simulink model "modelo_mpc_sem_restricao"  (R2018b)
settings: Solver=VariableStepAuto  StartTime=0.0  StopTime=100  RelTol=1e-3
values from neighbouring files (symbols this model uses):
  A = [0 1 0 0 ... (first row only)    [dadosBallBeam.m]    (also in dadosTanqueQuatro.m = [-1/T1 0 A3/(A1*T3) 0; tanqueQuatroLinearizacao.m = double(subs(As,{h1,h2,h3,h4,v1,v2},{h10,h20,h30,h40,v10,v20})
  A1 = 28    [dadosTanqueQuatro.m]    (also in tanqueQuatroLinearizacao.m)
  a1 = 0.071    [dadosTanqueQuatro.m]    (also in tanqueQuatroLinearizacao.m)
  A2 = 32    [dadosTanqueQuatro.m]    (also in tanqueQuatroLinearizacao.m)
  a2 = 0.057    [dadosTanqueQuatro.m]    (also in tanqueQuatroLinearizacao.m)
  a3 = 0.071    [dadosTanqueQuatro.m]    (also in tanqueQuatroLinearizacao.m)
  A3 = 28    [dadosTanqueQuatro.m]    (also in tanqueQuatroLinearizacao.m)
  a4 = 0.057    [dadosTanqueQuatro.m]    (also in tanqueQuatroLinearizacao.m)
  A4 = 32    [dadosTanqueQuatro.m]    (also in tanqueQuatroLinearizacao.m)
  B = [0 0 0 1]'    [dadosBallBeam.m]    (also in dadosTanqueQuatro.m = [(y1*k1)/A1 0; tanqueQuatroLinearizacao.m = double(subs(Bs,{h1,h2,h3,h4,v1,v2},{h10,h20,h30,h40,v10,v20})
  C = [1 0 0 0]    [dadosBallBeam.m]    (also in dadosTanqueQuatro.m = [1 0 0 0; tanqueQuatroLinearizacao.m = [1 0 0 0)
  D = [0]    [dadosBallBeam.m]    (also in dadosTanqueQuatro.m = [0 0; tanqueQuatroLinearizacao.m = [0 0)
  g = -9.8    [dadosBallBeam.m]    (also in dadosTanqueQuatro.m = 981; tanqueQuatroLinearizacao.m = 981)
  h1 = 12.4    [dadosTanqueQuatro.m]
  h2 = 12.7    [dadosTanqueQuatro.m]
  h3 = 1.8    [dadosTanqueQuatro.m]
  h4 = 1.4    [dadosTanqueQuatro.m]
  k1 = 3.33    [dadosTanqueQuatro.m]    (also in tanqueQuatroLinearizacao.m)
  k2 = 3.35    [dadosTanqueQuatro.m]    (also in tanqueQuatroLinearizacao.m)
  Kmpc = Kmpc(1:n_entradas,:)    [MPC_sem_restricao.m]    (also in dados_MPC_com_restricao.m; dados_MPC_com_restricao_estimador.m; dados_MPC_sem_restricao.m; dados_MPC_sem_restricao_estimador.m)
  Rl = Cp*Ap    [MPC_sem_restricao.m]    (also in dados_MPC_com_restricao.m; dados_MPC_com_restricao_estimador.m; dados_MPC_sem_restricao.m; dados_MPC_sem_restricao_estimador.m)
  ts = 0.1    [dados_MPC_com_restricao.m]    (also in dados_MPC_com_restricao_estimador.m; dados_MPC_sem_restricao.m; dados_MPC_sem_restricao_estimador.m)
  v1 = 3    [dadosTanqueQuatro.m]
  v2 = 3    [dadosTanqueQuatro.m]
  Wr = [Wr; eye(n_entradas)]    [MPC_sem_restricao.m]    (also in dados_MPC_com_restricao.m; dados_MPC_com_restricao_estimador.m; dados_MPC_sem_restricao.m; dados_MPC_sem_restricao_estimador.m)
  y1 = 0.7    [dadosTanqueQuatro.m]
  y2 = 0.6    [dadosTanqueQuatro.m]
undefined symbols (not defined in the file or in its folder): DiscIntNeverNeededParam
libraries: simulink x2
settings Model: Creator=Caléo  LastModifiedBy=Caléo

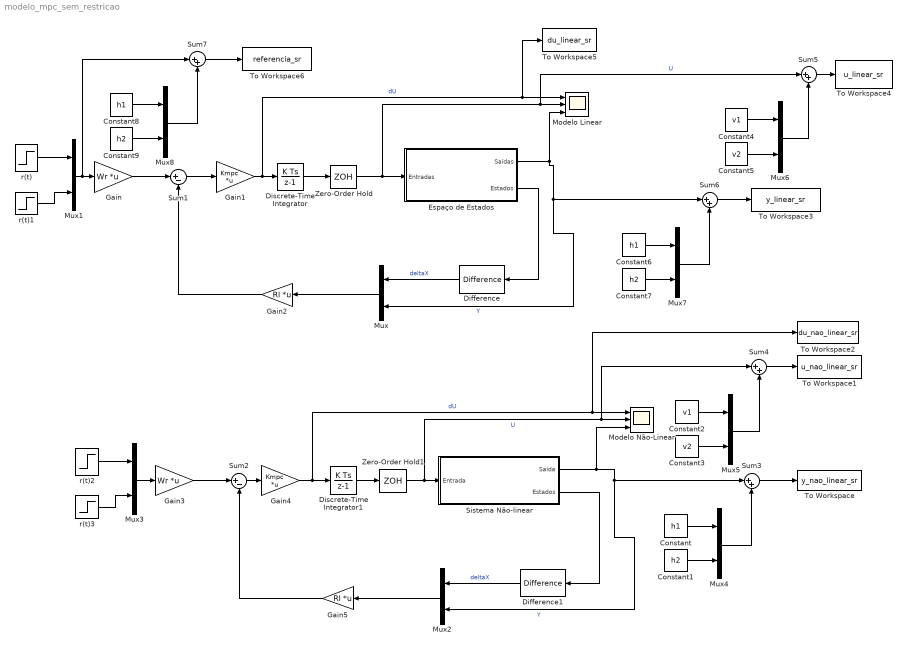
== system modelo_mpc_sem_restricao ==
  Constant : Constant  Value=h1
  Constant1 : Constant  Value=h2
  Constant2 : Constant  Value=v1
  Constant3 : Constant  Value=v2
  Constant4 : Constant  Value=v1
  Constant5 : Constant  Value=v2
  Constant6 : Constant  Value=h1
  Constant7 : Constant  Value=h2
  Constant8 : Constant  Value=h1
  Constant9 : Constant  Value=h2
  Difference : simulink/Discrete/Difference  ICPrevInput=0.0  OutMin=[]  OutMax=[]  OutDataType=fixdt(1, 16)  OutScaling=2^-10  DoSatur=off
  Difference1 : simulink/Discrete/Difference  ICPrevInput=0.0  OutMin=[]  OutMax=[]  OutDataType=fixdt(1, 16)  OutScaling=2^-10  DoSatur=off
  Discrete-Time Integrator : DiscreteIntegrator  SampleTime=ts  ICPrevOutput=DiscIntNeverNeededParam  ICPrevScaledInput=DiscIntNeverNeededParam
  Discrete-Time Integrator1 : DiscreteIntegrator  SampleTime=ts  ICPrevOutput=DiscIntNeverNeededParam  ICPrevScaledInput=DiscIntNeverNeededParam
  Espaço de Estados : Subsystem
  Gain : Gain  Gain=Wr  Multiplication=Matrix(K*u)
  Gain1 : Gain  Gain=Kmpc  Multiplication=Matrix(K*u)
  Gain2 : Gain  Gain=Rl  Multiplication=Matrix(K*u)
  Gain3 : Gain  Gain=Wr  Multiplication=Matrix(K*u)
  Gain4 : Gain  Gain=Kmpc  Multiplication=Matrix(K*u)
  Gain5 : Gain  Gain=Rl  Multiplication=Matrix(K*u)
  Modelo Linear : Scope  NumInputPorts=3
  Modelo Não-Linear : Scope  NumInputPorts=3
  Mux{,1..8} (9 alike) : Mux  Inputs=2
  Sistema Não-linear : Subsystem
  Sum1 : Sum  Inputs=|+-
  Sum2 : Sum  Inputs=|+-
  Sum{3..7} (5 alike) : Sum  Inputs=|++
  To Workspace : ToWorkspace  VariableName=y_nao_linear_sr  SaveFormat=Timeseries  SampleTime=-1
  To Workspace1 : ToWorkspace  VariableName=u_nao_linear_sr  SaveFormat=Timeseries  SampleTime=-1
  To Workspace2 : ToWorkspace  VariableName=du_nao_linear_sr  SaveFormat=Timeseries  SampleTime=-1
  To Workspace3 : ToWorkspace  VariableName=y_linear_sr  SaveFormat=Timeseries  SampleTime=-1
  To Workspace4 : ToWorkspace  VariableName=u_linear_sr  SaveFormat=Timeseries  SampleTime=-1
  To Workspace5 : ToWorkspace  VariableName=du_linear_sr  SaveFormat=Timeseries  SampleTime=-1
  To Workspace6 : ToWorkspace  VariableName=referencia_sr  SaveFormat=Timeseries  SampleTime=-1
  Zero-Order Hold : ZeroOrderHold  SampleTime=ts
  Zero-Order Hold1 : ZeroOrderHold  SampleTime=ts
  r(t) : Step  Time=0  After=2  SampleTime=0
  r(t)1 : Step  Time=0  After=-0.5  SampleTime=0
  r(t)2 : Step  Time=0  After=2  SampleTime=0
  r(t)3 : Step  Time=0  After=-0.5  SampleTime=0
  wires:
  Discrete-Time Integrator/1 -> Zero-Order Hold/1
  Espaço de Estados/1(Saídas) -> Modelo Linear/3, Mux/2, Sum6/1  "Y"
  Difference/1 -> Mux/1  "deltaX"
  Mux/1 -> Gain2/1
  Gain2/1 -> Sum1/2
  Gain1/1 -> To Workspace5/1, Modelo Linear/1, Discrete-Time Integrator/1  "dU"
  Sum1/1 -> Gain1/1
  Gain/1 -> Sum1/1
  Mux1/1 -> Sum7/1, Gain/1
  r(t)/1 -> Mux1/1
  r(t)1/1 -> Mux1/2
  Espaço de Estados/2(Estados) -> Difference/1
  Sistema Não-linear/2("Estados ") -> Difference1/1
  Mux2/1 -> Gain5/1
  Zero-Order Hold1/1 -> Sum4/1, Modelo Não-Linear/2, Sistema Não-linear/1(Entrada)  "U"
  r(t)2/1 -> Mux3/1
  Gain3/1 -> Sum2/1
  r(t)3/1 -> Mux3/2
  Mux3/1 -> Gain3/1
  Gain5/1 -> Sum2/2
  Sistema Não-linear/1("Saída ") -> Modelo Não-Linear/3, Sum3/1, Mux2/2  "Y"
  Gain4/1 -> To Workspace2/1, Modelo Não-Linear/1, Discrete-Time Integrator1/1  "dU"
  Discrete-Time Integrator1/1 -> Zero-Order Hold1/1
  Difference1/1 -> Mux2/1  "deltaX"
  Sum2/1 -> Gain4/1
  Zero-Order Hold/1 -> Sum5/1, Modelo Linear/2, Espaço de Estados/1(Entradas)  "U"
  Constant/1 -> Mux4/1
  Constant1/1 -> Mux4/2
  Sum3/1 -> To Workspace/1
  Mux4/1 -> Sum3/2
  Sum4/1 -> To Workspace1/1
  Mux5/1 -> Sum4/2
  Constant2/1 -> Mux5/1
  Constant3/1 -> Mux5/2
  Mux6/1 -> Sum5/2
  Constant5/1 -> Mux6/2
  Constant4/1 -> Mux6/1
  Sum5/1 -> To Workspace4/1
  Mux7/1 -> Sum6/2
  Constant6/1 -> Mux7/1
  Constant7/1 -> Mux7/2
  Sum6/1 -> To Workspace3/1
  Constant8/1 -> Mux8/1
  Constant9/1 -> Mux8/2
  Mux8/1 -> Sum7/2
  Sum7/1 -> To Workspace6/1

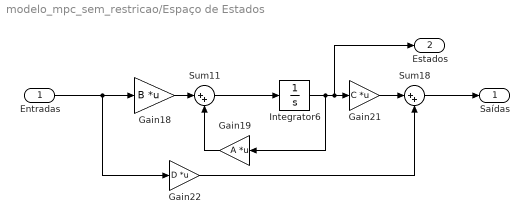
== system modelo_mpc_sem_restricao/Espaço de Estados ==
  Entradas : Inport
  Gain18 : Gain  Gain=B  Multiplication=Matrix(K*u)
  Gain19 : Gain  Gain=A  Multiplication=Matrix(K*u)
  Gain21 : Gain  Gain=C  Multiplication=Matrix(K*u)
  Gain22 : Gain  Gain=D  Multiplication=Matrix(K*u)
  Integrator6 : Integrator
  Sum11 : Sum  Inputs=|++
  Sum18 : Sum  Inputs=|++
  Saídas : Outport
  Estados : Outport  Port=2
  wires:
  Entradas/1 -> Gain22/1, Gain18/1
  Sum18/1 -> Saídas/1
  Gain22/1 -> Sum18/2
  Gain18/1 -> Sum11/1
  Gain19/1 -> Sum11/2
  Integrator6/1 -> Gain19/1, Estados/1, Gain21/1
  Sum11/1 -> Integrator6/1
  Gain21/1 -> Sum18/1

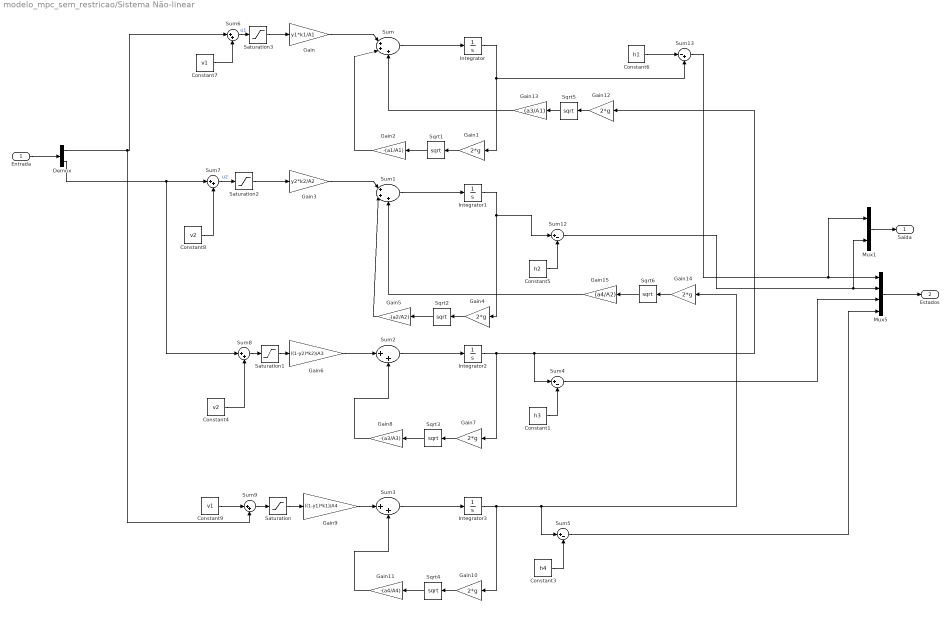
== system modelo_mpc_sem_restricao/Sistema Não-linear ==
  Entrada : Inport
  Constant1 : Constant  Value=h3
  Constant3 : Constant  Value=h4
  Constant4 : Constant  Value=v2
  Constant5 : Constant  Value=h2
  Constant6 : Constant  Value=h1
  Constant7 : Constant  Value=v1
  Constant8 : Constant  Value=v2
  Constant9 : Constant  Value=v1
  Demux : Demux  Outputs=2
  Gain : Gain  Gain=y1*k1/A1
  Gain{1,4,7,10,12,14} (6 alike) : Gain  Gain=2*g
  Gain11 : Gain  Gain=-(a4/A4)
  Gain13 : Gain  Gain=(a3/A1)
  Gain15 : Gain  Gain=(a4/A2)
  Gain2 : Gain  Gain=-(a1/A1)
  Gain3 : Gain  Gain=y2*k2/A2
  Gain5 : Gain  Gain=-(a2/A2)
  Gain6 : Gain  Gain=((1-y2)*k2)/A3
  Gain8 : Gain  Gain=-(a3/A3)
  Gain9 : Gain  Gain=((1-y1)*k1)/A4
  Integrator : Integrator  InitialCondition=h1  LimitOutput=on  UpperSaturationLimit=20  LowerSaturationLimit=0
  Integrator1 : Integrator  InitialCondition=h2  LimitOutput=on  UpperSaturationLimit=20  LowerSaturationLimit=0
  Integrator2 : Integrator  InitialCondition=h3  LimitOutput=on  UpperSaturationLimit=20  LowerSaturationLimit=0
  Integrator3 : Integrator  InitialCondition=h4  LimitOutput=on  UpperSaturationLimit=20  LowerSaturationLimit=0
  Mux1 : Mux  Inputs=2
  Mux5 : Mux
  Saturation{,1..3} (4 alike) : Saturate  UpperLimit=12  LowerLimit=0
  Sqrt{1..6} (6 alike) : Sqrt  SaturateOnIntegerOverflow=on
  Sum : Sum  Inputs=|+++
  Sum1 : Sum  Inputs=|+++
  Sum12 : Sum  Inputs=|+-
  Sum13 : Sum  Inputs=|-+
  Sum{2..3,6..9} (6 alike) : Sum  Inputs=|++
  Sum4 : Sum  Inputs=|+-
  Sum5 : Sum  Inputs=|+-
  "Saída " : Outport
  "Estados " : Outport  Port=2
  wires:
  Demux/1 -> Sum9/2, Sum6/1
  Demux/2 -> Sum8/1, Sum7/1
  Mux1/1 -> "Saída "/1
  Constant9/1 -> Sum9/1
  Sum8/1 -> Saturation1/1
  Entrada/1 -> Demux/1
  Sum5/1 -> Mux5/4
  Sum13/1 -> Mux1/1, Mux5/1
  Gain8/1 -> Sum2/2
  Sqrt5/1 -> Gain13/1
  Gain12/1 -> Sqrt5/1
  Integrator3/1 -> Sum5/1, Gain14/1, Gain10/1
  Saturation3/1 -> Gain/1
  Sqrt2/1 -> Gain5/1
  Integrator2/1 -> Sum4/1, Gain12/1, Gain7/1
  Constant6/1 -> Sum13/1
  Sum4/1 -> Mux5/3
  Sqrt1/1 -> Gain2/1
  Gain9/1 -> Sum3/1
  Gain14/1 -> Sqrt6/1
  Sum3/1 -> Integrator3/1
  Gain/1 -> Sum/1
  Gain7/1 -> Sqrt3/1
  Gain13/1 -> Sum/3
  Constant8/1 -> Sum7/2
  Integrator/1 -> Sum13/2, Gain1/1
  Gain6/1 -> Sum2/1
  Saturation1/1 -> Gain6/1
  Saturation/1 -> Gain9/1
  Sqrt6/1 -> Gain15/1
  Constant1/1 -> Sum4/2
  Constant7/1 -> Sum6/2
  Integrator1/1 -> Gain4/1, Sum12/1
  Sqrt4/1 -> Gain11/1
  Sum6/1 -> Saturation3/1  "u1"
  Sqrt3/1 -> Gain8/1
  Gain2/1 -> Sum/2
  Sum2/1 -> Integrator2/1
  Gain5/1 -> Sum1/2
  Gain3/1 -> Sum1/1
  Sum7/1 -> Saturation2/1  "u2"
  Gain1/1 -> Sqrt1/1
  Mux5/1 -> "Estados "/1
  Sum1/1 -> Integrator1/1
  Sum12/1 -> Mux1/2, Mux5/2
  Gain4/1 -> Sqrt2/1
  Gain11/1 -> Sum3/2
  Sum/1 -> Integrator/1
  Constant5/1 -> Sum12/2
  Gain15/1 -> Sum1/3
  Gain10/1 -> Sqrt4/1
  Constant4/1 -> Sum8/2
  Constant3/1 -> Sum5/2
  Sum9/1 -> Saturation/1
  Saturation2/1 -> Gain3/1
